simulink model "FOC_Host_Site2"  (R2025b)
settings: Solver=FixedStepDiscrete  StartTime=0.0  StopTime=inf  RelTol=1e-3  EnableMultiTasking=on
values from neighbouring files (symbols this model uses):
  Ts = T_pwm    (= 5e-05)    [FOC_Motor_Control_Params.m]    (also in mcb_pmsm_foc_qep_f28069LaunchPad_data.m)
libraries: instrumentseriallib x3

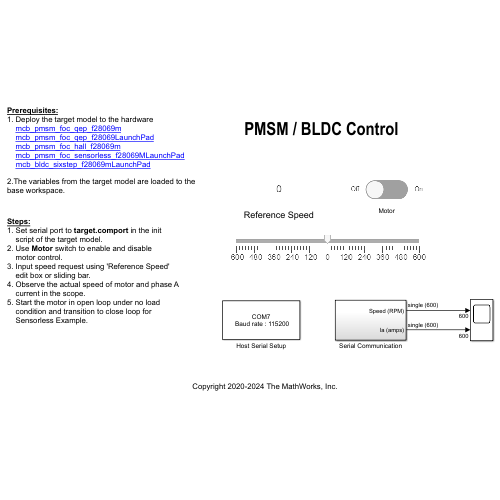
[thumbnail: Simulink's stored preview of the top-level diagram]
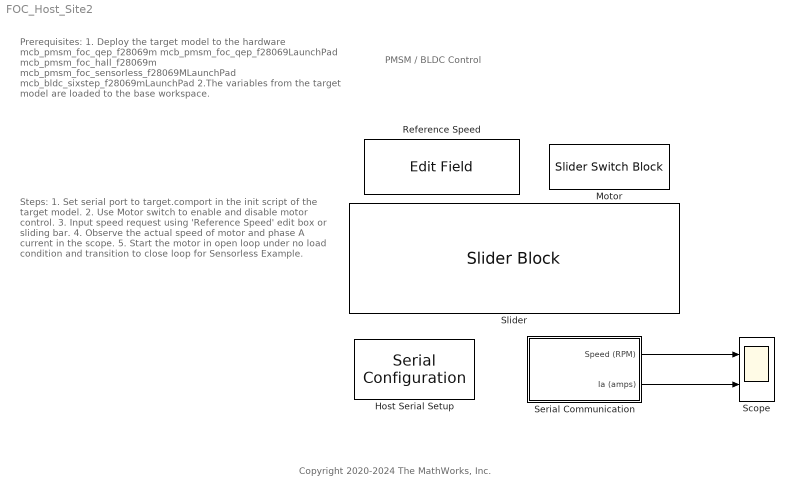
== system FOC_Host_Site2 ==
  note: Copyright 2020-2024 The MathWorks, Inc.
  note: Steps:
      | 1. Set serial port to target.comport in the init
      | script of the target model.
      | 2. Use Motor switch to enable and disable
      | motor control.
      | 3. Input speed request using 'Reference Speed'
      | edit box or sliding bar.
      | 4. Observe the actual speed of motor and phase A
      | current in the scope.
      | 5. Start the motor in open loop under no load
      | condition and transition to close loop for
      | Sensorless Example.
  note: PMSM / BLDC Control
  note: Prerequisites:
      | 1. Deploy the target model to the hardware
      | mcb_pmsm_foc_qep_f28069m
      | mcb_pmsm_foc_qep_f28069LaunchPad
      | mcb_pmsm_foc_hall_f28069m
      | mcb_pmsm_foc_sensorless_f28069MLaunchPad
      | mcb_bldc_sixstep_f28069mLaunchPad
      |
      | 2.The variables from the target model are loaded to the base workspace.
  Host Serial Setup : instrumentseriallib/Serial Configuration  Priority=-99  PortSel=target.comport  Port=target.comport  ComPort=target.comport  BaudRate=115200  DataBits=8  Parity=none  StopBits=1  ByteOrder=little-endian  FlowControl=none  Timeout=2  SimulateUsing=Interpreted execution  BlockInModel=on  aMode=5
  Motor : SliderSwitchBlock  LabelPosition=Hide
  Reference Speed : EditField  LabelPosition=Hide  ShowInitialText=on  Alignment=Center
  Scope : Scope  NumInputPorts=2
  Serial Communication : Subsystem
  Slider : SliderBlock  LabelPosition=Hide  ScaleMin=-600  ScaleMax=600
  wires:
  Serial Communication/1(Speed (RPM)) -> Scope/1
  Serial Communication/2(Ia (amps)) -> Scope/2

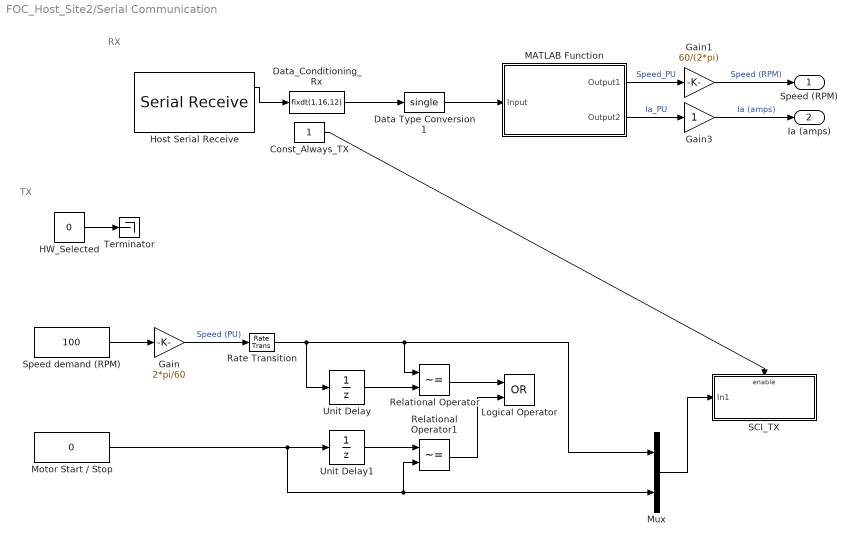
== system FOC_Host_Site2/Serial Communication ==
  note: RX
  note: TX
  Const_Always_TX : Constant  OutDataTypeStr=boolean
  Data Type Conversion1 : DataTypeConversion  OutDataTypeStr=single  RndMeth=Simplest  SaturateOnIntegerOverflow=off
  Data_Conditioning_Rx : DataTypeConversion  OutDataTypeStr=fixdt(1,16,12)  ConvertRealWorld=Stored Integer (SI)  RndMeth=Simplest  SaturateOnIntegerOverflow=off
  Gain : Gain  Gain=2*pi/60  RndMeth=Simplest  OutDataTypeStr=Inherit: Same as input
  Gain1 : Gain  Gain=60/(2*pi)  OutDataTypeStr=single  RndMeth=Simplest
  Gain3 : Gain  OutDataTypeStr=single  RndMeth=Simplest
  HW_Selected : Constant  Value=0  OutDataTypeStr=uint8
  Host Serial Receive : instrumentseriallib/Serial Receive  PortSel=target.comport  Port=target.comport  ComPort=target.comport  DataType=single  SaveDataType=uint8  ToggleHeader=on  Header='S'  ToggleDataSize=on  DataSize=[1 2]  ToggleTerminator=on  Terminator=Custom terminator  CustomTerminator='E'  InputFormat=Row major  EnableBlockingMode=off  ActionDataUnavailable=Output last received value  ActionWhenDataUnavailable=Output last received value  CustomValue=0  SampleTime=600 * Ts  SimulateUsing=Interpreted execution  BlockInModel=on  aMode=5  LibraryInUse=instrumentlib
  Logical Operator : Logic  Operator=OR  AllPortsSameDT=off  OutDataTypeStr=boolean
  MATLAB Function : MATLAB Function  TreatAsAtomicUnit=on
  Motor Start / Stop : Constant  Value=0  VectorParams1D=off  OutDataTypeStr=single  SampleTime=0.03
  Mux : Mux  Inputs=2
  Rate Transition : RateTransition  OutPortSampleTime=0.03
  Relational Operator : RelationalOperator  Operator=~=  OutDataTypeStr=boolean  InputSameDT=off
  Relational Operator1 : RelationalOperator  Operator=~=  OutDataTypeStr=boolean  InputSameDT=off
  SCI_TX : Subsystem  TreatAsAtomicUnit=on
  Speed demand (RPM) : Constant  Value=100  VectorParams1D=off  OutDataTypeStr=single  SampleTime=0.03
  Terminator : Terminator
  Unit Delay : UnitDelay  InitialCondition=0.5  SampleTime=-1  HasFrameUpgradeWarning=on
  Unit Delay1 : UnitDelay  SampleTime=-1  HasFrameUpgradeWarning=on
  Speed (RPM) : Outport
  Ia (amps) : Outport  Port=2
  wires:
  HW_Selected/1 -> Terminator/1
  Unit Delay1/1 -> Relational Operator1/1
  Relational Operator1/1 -> Logical Operator/2
  Unit Delay/1 -> Relational Operator/2
  Relational Operator/1 -> Logical Operator/1
  Gain/1 -> Rate Transition/1  "Speed (PU)"
  Speed demand (RPM)/1 -> Gain/1
  Mux/1 -> SCI_TX/1(In1)
  Rate Transition/1 -> Unit Delay/1, Mux/1, Relational Operator/1
  Motor Start / Stop/1 -> Relational Operator1/2, Mux/2, Unit Delay1/1
  MATLAB Function/2(Output2) -> Gain3/1  "Ia_PU"
  Gain3/1 -> Ia (amps)/1  "Ia (amps)"
  Host Serial Receive/1 -> Data_Conditioning_Rx/1
  MATLAB Function/1(Output1) -> Gain1/1  "Speed_PU"
  Gain1/1 -> Speed (RPM)/1  "Speed (RPM)"
  Data_Conditioning_Rx/1 -> Data Type Conversion1/1
  Data Type Conversion1/1 -> MATLAB Function/1(Input)
  Const_Always_TX/1 -> SCI_TX/Enable

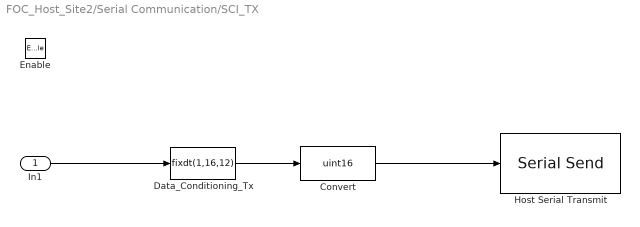
== system FOC_Host_Site2/Serial Communication/SCI_TX ==
  In1 : Inport
  Enable : EnablePort
  Convert : DataTypeConversion  OutDataTypeStr=uint16  ConvertRealWorld=Stored Integer (SI)  RndMeth=Simplest  SaturateOnIntegerOverflow=off
  Data_Conditioning_Tx : DataTypeConversion  OutDataTypeStr=fixdt(1,16,12)  RndMeth=Simplest  SaturateOnIntegerOverflow=off
  Host Serial Transmit : instrumentseriallib/Serial Send  PortSel=target.comport  Port=target.comport  ComPort=target.comport  Header='S'  Terminator=Custom terminator  CustomTerminator='E'  EnableBlockingMode=off  SimulateUsing=Interpreted execution  BlockInModel=on  aMode=5
  wires:
  Convert/1 -> Host Serial Transmit/1
  Data_Conditioning_Tx/1 -> Convert/1
  In1/1 -> Data_Conditioning_Tx/1

== matlab function FOC_Host_Site2/Serial Communication/MATLAB Function ==
function [ Output1, Output2] = unBuf(Input)

Output1 = Input(:, 1);
Output2 = Input(:, 2);
end
